simulink library "downlink_4c2t_cordic_lib"  (Simulink 8.7)
settings: Solver=ode45  StartTime=0.0  StopTime=10.0  RelTol=1e-3
undefined symbols (not defined in the file or in its folder): evalAionMaskParam, primtype, value
undefined symbols (not defined in the file): nco_angle_bits, nco_out_bits
libraries: DSPBAPrim x55, CORDIC_lib x35
settings Model: Creator=bcope  LastModifiedBy=5g

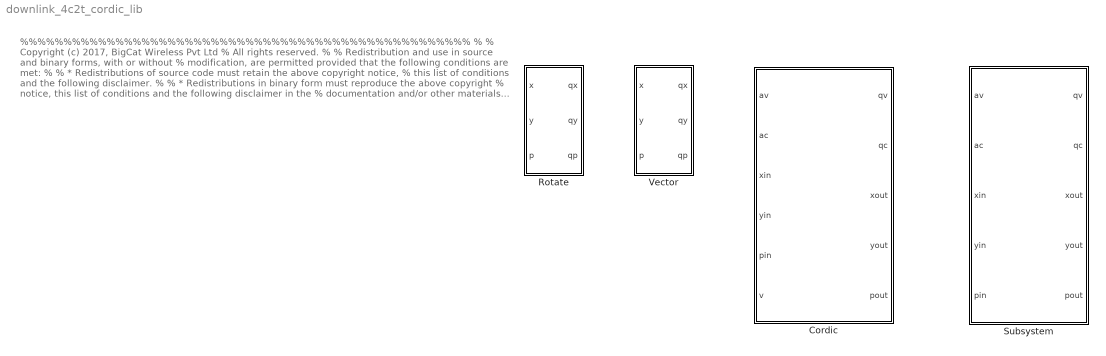
== system downlink_4c2t_cordic_lib ==
  note: %%%%%%%%%%%%%%%%%%%%%%%%%%%%%%%%%%%%%%%%%%%%%%%%%%%%
      |  %
      |  % Copyright (c) 2017, BigCat Wireless Pvt Ltd
      |  % All rights reserved.
      |  %
      |  % Redistribution and use in source and binary forms, with or without
      |  % modification, are permitted provided that the following conditions are met:
      |  %
      |  %     * Redistributions of source code must retain the above copyright notice,
      |  %       this list of conditions and the following disclaimer.
      |  %
      |  %     * Redistributions in binary form must reproduce the above copyright
      |  %       notice, this list of conditions and the following disclaimer in the
      |  %       documentation and/or other materials provided with the distribution.
      |  %
      |  %     * Neither the name of the copyright holder nor the names of its contributors
      |  %       may be used to endorse or promote products derived from this software
      |  %       without specific prior written permission.
      |  %
      |  %
      |  %
      |  % THIS SOFTWARE IS PROVIDED BY THE COPYRIGHT HOLDERS AND CONTRIBUTORS "AS IS"
      |  % AND ANY EXPRESS OR IMPLIED WARRANTIES, INCLUDING, BUT NOT LIMITED TO, THE
      |  % IMPLIED WARRANTIES OF MERCHANTABILITY AND FITNESS FOR A PARTICULAR PURPOSE ARE
      |  % DISCLAIMED. IN NO EVENT SHALL THE COPYRIGHT HOLDER OR CONTRIBUTORS BE LIABLE
      |  % FOR ANY DIRECT, INDIRECT, INCIDENTAL, SPECIAL, EXEMPLARY, OR CONSEQUENTIAL
      |  % DAMAGES (INCLUDING, BUT NOT LIMITED TO, PROCUREMENT OF SUBSTITUTE GOODS OR
      |  % SERVICES; LOSS OF USE, DATA, OR PROFITS; OR BUSINESS INTERRUPTION) HOWEVER
      |  % CAUSED AND ON ANY THEORY OF LIABILITY, WHETHER IN CONTRACT, STRICT LIABILITY,
      |  % OR TORT (INCLUDING NEGLIGENCE OR OTHERWISE) ARISING IN ANY WAY OUT OF THE USE
      |  % OF THIS SOFTWARE, EVEN IF ADVISED OF THE POSSIBILITY OF SUCH DAMAGE.
      |  %
      |   %%%%%%%%%%%%%%%%%%%%%%%%%%%%%%%%%%%%%%%%%%%%%%%%%%%%%
  Cordic : Subsystem  mask(CORDIC range -pi/2 to pi/2){stages=16, angle_bits=16, angle_frac_bits=14, xy_bits=16, xy_frac_bits=14}
      mask prompts: angle_bits "Angle bits"; angle_frac_bits "Angle fractional bits"; xy_bits "XY bits"; xy_frac_bits "XY fractional bits"
      mask help:
      | Primitive block implementation of CORDIC.
      | Range -pi/2 to pi/2
      |
      | See "Help" for information on parameter selection.
      mask init:
      | setup_cordic_block(stages, angle_bits, angle_frac_bits, xy_bits, xy_frac_bits);
      mask Help:
      | By default it is expected that stages = angle_bits = xy_bits also that
      | angle_frac_bits = angle_bits-2 (i.e. 2 integer angle bits)
      | 
      | It is assumed that stages <= angle_bits and stages <= xy_bits
      | 
      | Parameter description:
      | 
      | Stages (stages)
      | Number of CORDIC stages
      | Note counting starts at zero so "iterations = stages+1"
      | 
      | Angle bits (angle_bits)
      | Number of bits used to represent the angle, data format is "sfix"
      | 
      | Angle fractional bits (angle_frac_bits)
      | Number of angle bits which are fractional
      | Angle format will be "sfix[angle_bits]_[angle_frac_bits]"
      | 
      | XY bits (xy_bits)
      | Number of bits used to represent inputs x,y, data format is "sfix"
      | 
      | XY fractional bits (xy_frac_bits)
      | Number of x,y bits which are fractional
      | Format will be "sfix[xy_bits]_[xy_frac_bits]"
      | 
      | 
      | For more information on CORDIC see the following paper (from which this
      | implementation was created):
      | 
      | "A survey of CORDIC algorithms for FPGAs"
      | Ray Andraka, FPGA '98
      mask Display:
      | % calculate gain
      | gain = 1;
      | for i=0:stages
      |     gain = gain*(sqrt((1+2^(-2*i))));
      | end
      | color('w');image(imread('dspba_prim.jpg'));
      | fprintf('CORDIC\n(pi/2 to -pi/2)\ngain=%1.4f\niterations=%i',gain,stages+1);
      | 
      | port_label('input',1,'v_in');
      | port_label('input',2,'c_in');
      | port_label('input',3,'x_in');
      | port_label('input',4,'y_in');
      | port_label('input',5,'p_in');
      | port_label('input',6,'mode');
      | port_label('output',1,'v_out');
      | port_label('output',2,'c_out');
      | port_label('output',3,'x_out');
      | port_label('output',4,'y_out');
      | port_label('output',5,'p_out');
  Rotate : Subsystem  mask{stage=0, angle_bits=16, angle_frac_bits=14, xy_bits=16, xy_frac_bits=14}
      mask prompts: angle_bits "Angle bit width"; angle_frac_bits "Angle fractional bits"; xy_bits "XY bit width"; xy_frac_bits "XY fractional bits"
  Subsystem : Subsystem  mask{stages=nco_angle_bits, angle_bits=nco_angle_bits, angle_frac_bits=nco_angle_bits-3, xy_bits=nco_out_bits, xy_frac_bits=nco_out_bits-2}
      mask prompts: angle_bits "Angle bits"; angle_frac_bits "Angle fractional bits"; xy_bits "XY bits"; xy_frac_bits "XY fractional bits"
      mask init:
      | sys = gcb;
      | 
      | % error trapping
      | if (angle_bits-angle_frac_bits)<3
      |     fprintf(['Warning (' sys ') not sufficient angle integer bits to represent full angle swing (-pi to pi)']);
      | end
      | 
      | if angle_bits < stages 
      |     fprintf(['Warning (' sys ') #angle bits < stages behaviour may be unexpected']);
      | end
      | 
      | if xy_bits < stages 
      |     fprintf(['Warning (' sys ') #xy bits < stages behaviour may be unexpected']);
      | end
      mask Display:
      | % calculate gain
      | gain = 1;
      | for i=0:stages
      |     gain = gain*(sqrt((1+2^(-2*i))));
      | end
      | color('w');image(imread('dspba_prim.jpg'));
      | fprintf('CORDIC\nRotate\n(pi to -pi)\ngain=%1.4f\niterations=%i',gain,stages+1);
      | port_label('input',1,'v_in');
      | port_label('input',2,'c_in');
      | port_label('input',3,'x_in');
      | port_label('input',4,'y_in');
      | port_label('input',5,'p_in');
      | port_label('output',1,'v_out');
      | port_label('output',2,'c_out');
      | port_label('output',3,'x_out');
      | port_label('output',4,'y_out');
      | port_label('output',5,'p_out');
  Vector : Subsystem  mask{stage=0, angle_bits=16, angle_frac_bits=14, xy_bits=16, xy_frac_bits=14}
      mask prompts: angle_bits "Angle bits"; angle_frac_bits "Angle fractional bits"; xy_bits "XY bits"; xy_frac_bits "XY fractional bits"

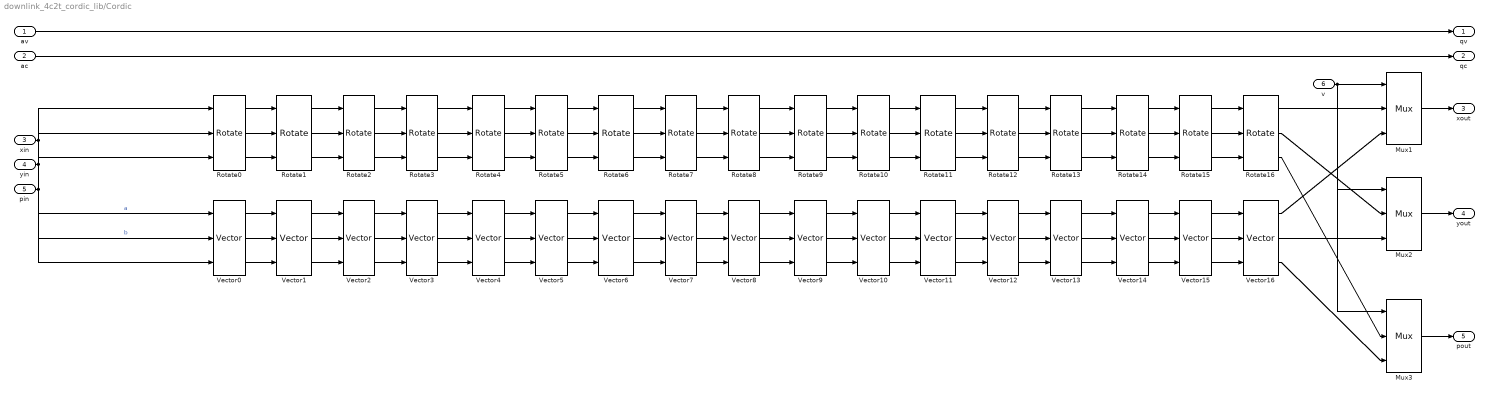
== system downlink_4c2t_cordic_lib/Cordic ==
  av : Inport
  ac : Inport  Port=2
  xin : Inport  Port=3
  yin : Inport  Port=4
  pin : Inport  Port=5
  v : Inport  Port=6
  Mux1 : DSPBAPrim/Mux  primtype=mux  nInputs=evalAionMaskParam(gcb,'value',1)+1  nOutputs=1  omode=Inherit via internal rule  otype=sfix(16)  scale=2^-15  rndmethod=Unbiased  factor=1  satmethod=Symmetric  shift_vec=[0 1 2 -1]  value=2  inPortNames=['s'; 'd0'; 'd1'; 'd2'; 'd3'; 'd4'; 'd5'; 'd6'; 'd7'; 'd8'; 'd9';]  outPortNames=[' ']  dspbaimage=dspba_prim.jpg  text=fprintf('%s', primtype);  style=Optimised  visibilities=1032  version=20131025
  Mux2 : DSPBAPrim/Mux  primtype=mux  nInputs=evalAionMaskParam(gcb,'value',1)+1  nOutputs=1  omode=Inherit via internal rule  otype=sfix(16)  scale=2^-15  rndmethod=Unbiased  factor=1  satmethod=Symmetric  shift_vec=[0 1 2 -1]  value=2  inPortNames=['s'; 'd0'; 'd1'; 'd2'; 'd3'; 'd4'; 'd5'; 'd6'; 'd7'; 'd8'; 'd9';]  outPortNames=[' ']  dspbaimage=dspba_prim.jpg  text=fprintf('%s', primtype);  style=Optimised  visibilities=1032  version=20131025
  Mux3 : DSPBAPrim/Mux  primtype=mux  nInputs=evalAionMaskParam(gcb,'value',1)+1  nOutputs=1  omode=Inherit via internal rule  otype=sfix(16)  scale=2^-15  rndmethod=Unbiased  factor=1  satmethod=Symmetric  shift_vec=[0 1 2 -1]  value=2  inPortNames=['s'; 'd0'; 'd1'; 'd2'; 'd3'; 'd4'; 'd5'; 'd6'; 'd7'; 'd8'; 'd9';]  outPortNames=[' ']  dspbaimage=dspba_prim.jpg  text=fprintf('%s', primtype);  style=Optimised  visibilities=1032  version=20131025
  Rotate0 : CORDIC_lib/Rotate  stage=0  angle_bits=16  angle_frac_bits=14  xy_bits=16  xy_frac_bits=14
  Rotate1 : CORDIC_lib/Rotate  stage=1  angle_bits=16  angle_frac_bits=14  xy_bits=16  xy_frac_bits=14
  Rotate10 : CORDIC_lib/Rotate  stage=10  angle_bits=16  angle_frac_bits=14  xy_bits=16  xy_frac_bits=14
  Rotate11 : CORDIC_lib/Rotate  stage=11  angle_bits=16  angle_frac_bits=14  xy_bits=16  xy_frac_bits=14
  Rotate12 : CORDIC_lib/Rotate  stage=12  angle_bits=16  angle_frac_bits=14  xy_bits=16  xy_frac_bits=14
  Rotate13 : CORDIC_lib/Rotate  stage=13  angle_bits=16  angle_frac_bits=14  xy_bits=16  xy_frac_bits=14
  Rotate14 : CORDIC_lib/Rotate  stage=14  angle_bits=16  angle_frac_bits=14  xy_bits=16  xy_frac_bits=14
  Rotate15 : CORDIC_lib/Rotate  stage=15  angle_bits=16  angle_frac_bits=14  xy_bits=16  xy_frac_bits=14
  Rotate16 : CORDIC_lib/Rotate  stage=16  angle_bits=16  angle_frac_bits=14  xy_bits=16  xy_frac_bits=14
  Rotate2 : CORDIC_lib/Rotate  stage=2  angle_bits=16  angle_frac_bits=14  xy_bits=16  xy_frac_bits=14
  Rotate3 : CORDIC_lib/Rotate  stage=3  angle_bits=16  angle_frac_bits=14  xy_bits=16  xy_frac_bits=14
  Rotate4 : CORDIC_lib/Rotate  stage=4  angle_bits=16  angle_frac_bits=14  xy_bits=16  xy_frac_bits=14
  Rotate5 : CORDIC_lib/Rotate  stage=5  angle_bits=16  angle_frac_bits=14  xy_bits=16  xy_frac_bits=14
  Rotate6 : CORDIC_lib/Rotate  stage=6  angle_bits=16  angle_frac_bits=14  xy_bits=16  xy_frac_bits=14
  Rotate7 : CORDIC_lib/Rotate  stage=7  angle_bits=16  angle_frac_bits=14  xy_bits=16  xy_frac_bits=14
  Rotate8 : CORDIC_lib/Rotate  stage=8  angle_bits=16  angle_frac_bits=14  xy_bits=16  xy_frac_bits=14
  Rotate9 : CORDIC_lib/Rotate  stage=9  angle_bits=16  angle_frac_bits=14  xy_bits=16  xy_frac_bits=14
  Vector0 : CORDIC_lib/Vector  stage=0  angle_bits=16  angle_frac_bits=14  xy_bits=16  xy_frac_bits=14
  Vector1 : CORDIC_lib/Vector  stage=1  angle_bits=16  angle_frac_bits=14  xy_bits=16  xy_frac_bits=14
  Vector10 : CORDIC_lib/Vector  stage=10  angle_bits=16  angle_frac_bits=14  xy_bits=16  xy_frac_bits=14
  Vector11 : CORDIC_lib/Vector  stage=11  angle_bits=16  angle_frac_bits=14  xy_bits=16  xy_frac_bits=14
  Vector12 : CORDIC_lib/Vector  stage=12  angle_bits=16  angle_frac_bits=14  xy_bits=16  xy_frac_bits=14
  Vector13 : CORDIC_lib/Vector  stage=13  angle_bits=16  angle_frac_bits=14  xy_bits=16  xy_frac_bits=14
  Vector14 : CORDIC_lib/Vector  stage=14  angle_bits=16  angle_frac_bits=14  xy_bits=16  xy_frac_bits=14
  Vector15 : CORDIC_lib/Vector  stage=15  angle_bits=16  angle_frac_bits=14  xy_bits=16  xy_frac_bits=14
  Vector16 : CORDIC_lib/Vector  stage=16  angle_bits=16  angle_frac_bits=14  xy_bits=16  xy_frac_bits=14
  Vector2 : CORDIC_lib/Vector  stage=2  angle_bits=16  angle_frac_bits=14  xy_bits=16  xy_frac_bits=14
  Vector3 : CORDIC_lib/Vector  stage=3  angle_bits=16  angle_frac_bits=14  xy_bits=16  xy_frac_bits=14
  Vector4 : CORDIC_lib/Vector  stage=4  angle_bits=16  angle_frac_bits=14  xy_bits=16  xy_frac_bits=14
  Vector5 : CORDIC_lib/Vector  stage=5  angle_bits=16  angle_frac_bits=14  xy_bits=16  xy_frac_bits=14
  Vector6 : CORDIC_lib/Vector  stage=6  angle_bits=16  angle_frac_bits=14  xy_bits=16  xy_frac_bits=14
  Vector7 : CORDIC_lib/Vector  stage=7  angle_bits=16  angle_frac_bits=14  xy_bits=16  xy_frac_bits=14
  Vector8 : CORDIC_lib/Vector  stage=8  angle_bits=16  angle_frac_bits=14  xy_bits=16  xy_frac_bits=14
  Vector9 : CORDIC_lib/Vector  stage=9  angle_bits=16  angle_frac_bits=14  xy_bits=16  xy_frac_bits=14
  qv : Outport
  qc : Outport  Port=2
  xout : Outport  Port=3
  yout : Outport  Port=4
  pout : Outport  Port=5
  wires:
  av/1 -> qv/1
  ac/1 -> qc/1
  xin/1 -> Rotate0/1, Vector0/1  "a"
  yin/1 -> Rotate0/2, Vector0/2  "b"
  pin/1 -> Rotate0/3, Vector0/3
  Rotate0/1 -> Rotate1/1
  Vector0/1 -> Vector1/1
  Rotate0/2 -> Rotate1/2
  Vector0/2 -> Vector1/2
  Rotate0/3 -> Rotate1/3
  Vector0/3 -> Vector1/3
  Rotate1/1 -> Rotate2/1
  Vector1/1 -> Vector2/1
  Rotate1/2 -> Rotate2/2
  Vector1/2 -> Vector2/2
  Rotate1/3 -> Rotate2/3
  Vector1/3 -> Vector2/3
  Rotate2/1 -> Rotate3/1
  Vector2/1 -> Vector3/1
  Rotate2/2 -> Rotate3/2
  Vector2/2 -> Vector3/2
  Rotate2/3 -> Rotate3/3
  Vector2/3 -> Vector3/3
  Rotate3/1 -> Rotate4/1
  Vector3/1 -> Vector4/1
  Rotate3/2 -> Rotate4/2
  Vector3/2 -> Vector4/2
  Rotate3/3 -> Rotate4/3
  Vector3/3 -> Vector4/3
  Rotate4/1 -> Rotate5/1
  Vector4/1 -> Vector5/1
  Rotate4/2 -> Rotate5/2
  Vector4/2 -> Vector5/2
  Rotate4/3 -> Rotate5/3
  Vector4/3 -> Vector5/3
  Rotate5/1 -> Rotate6/1
  Vector5/1 -> Vector6/1
  Rotate5/2 -> Rotate6/2
  Vector5/2 -> Vector6/2
  Rotate5/3 -> Rotate6/3
  Vector5/3 -> Vector6/3
  Rotate6/1 -> Rotate7/1
  Vector6/1 -> Vector7/1
  Rotate6/2 -> Rotate7/2
  Vector6/2 -> Vector7/2
  Rotate6/3 -> Rotate7/3
  Vector6/3 -> Vector7/3
  Rotate7/1 -> Rotate8/1
  Vector7/1 -> Vector8/1
  Rotate7/2 -> Rotate8/2
  Vector7/2 -> Vector8/2
  Rotate7/3 -> Rotate8/3
  Vector7/3 -> Vector8/3
  Rotate8/1 -> Rotate9/1
  Vector8/1 -> Vector9/1
  Rotate8/2 -> Rotate9/2
  Vector8/2 -> Vector9/2
  Rotate8/3 -> Rotate9/3
  Vector8/3 -> Vector9/3
  Rotate9/1 -> Rotate10/1
  Vector9/1 -> Vector10/1
  Rotate9/2 -> Rotate10/2
  Vector9/2 -> Vector10/2
  Rotate9/3 -> Rotate10/3
  Vector9/3 -> Vector10/3
  Rotate10/1 -> Rotate11/1
  Vector10/1 -> Vector11/1
  Rotate10/2 -> Rotate11/2
  Vector10/2 -> Vector11/2
  Rotate10/3 -> Rotate11/3
  Vector10/3 -> Vector11/3
  Rotate11/1 -> Rotate12/1
  Vector11/1 -> Vector12/1
  Rotate11/2 -> Rotate12/2
  Vector11/2 -> Vector12/2
  Rotate11/3 -> Rotate12/3
  Vector11/3 -> Vector12/3
  Rotate12/1 -> Rotate13/1
  Vector12/1 -> Vector13/1
  Rotate12/2 -> Rotate13/2
  Vector12/2 -> Vector13/2
  Rotate12/3 -> Rotate13/3
  Vector12/3 -> Vector13/3
  Rotate13/1 -> Rotate14/1
  Vector13/1 -> Vector14/1
  Rotate13/2 -> Rotate14/2
  Vector13/2 -> Vector14/2
  Rotate13/3 -> Rotate14/3
  Vector13/3 -> Vector14/3
  Rotate14/1 -> Rotate15/1
  Vector14/1 -> Vector15/1
  Rotate14/2 -> Rotate15/2
  Vector14/2 -> Vector15/2
  Rotate14/3 -> Rotate15/3
  Vector14/3 -> Vector15/3
  Rotate15/1 -> Rotate16/1
  Vector15/1 -> Vector16/1
  Rotate15/2 -> Rotate16/2
  Vector15/2 -> Vector16/2
  Rotate15/3 -> Rotate16/3
  Vector15/3 -> Vector16/3
  v/1 -> Mux1/1, Mux2/1, Mux3/1
  Rotate16/1 -> Mux1/2
  Vector16/1 -> Mux1/3
  Rotate16/2 -> Mux2/2
  Vector16/2 -> Mux2/3
  Rotate16/3 -> Mux3/2
  Vector16/3 -> Mux3/3
  Mux1/1 -> xout/1
  Mux2/1 -> yout/1
  Mux3/1 -> pout/1

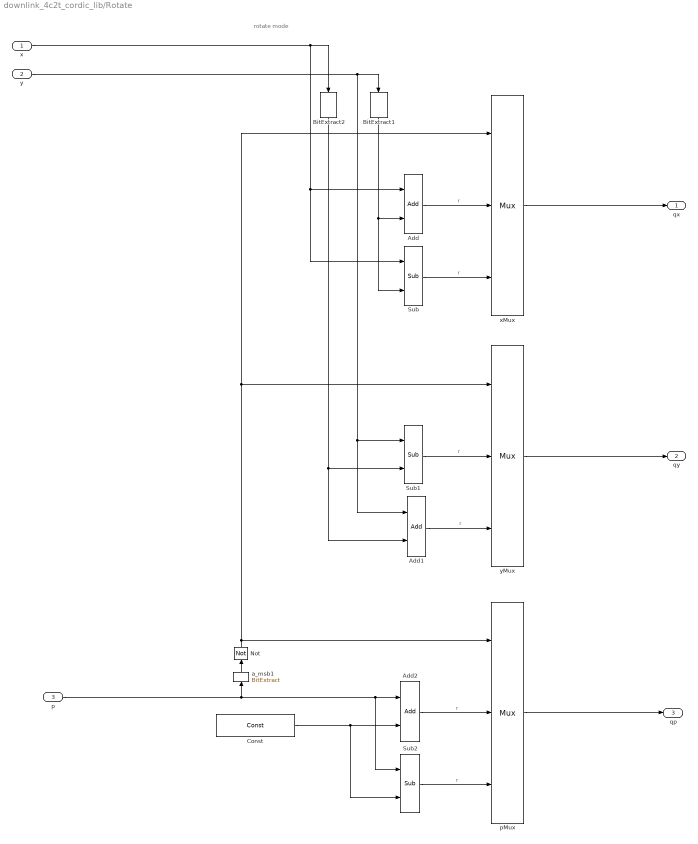
== system downlink_4c2t_cordic_lib/Rotate ==
  note: rotate mode
  x : Inport
  y : Inport  Port=2
  p : Inport  Port=3
  Add : DSPBAPrim/Add  primtype=add  nInputs=evalAionMaskParam(gcb,'value',1)  nOutputs=1  omode=Inherit via internal rule  otype=sfix(16)  scale=2^-15  rndmethod=Unbiased  factor=1  satmethod=Symmetric  shift_vec=[0 1 2 -1]  value=2  inPortNames=[' '; ' ';]  outPortNames=[' ']  dspbaimage=dspba_prim.jpg  text=fprintf('+');  style=Optimised  visibilities=1032  genFPC=off  floatRounding=correct  advOptions=[]  version=20130821
  Add1 : DSPBAPrim/Add  primtype=add  nInputs=evalAionMaskParam(gcb,'value',1)  nOutputs=1  omode=Inherit via internal rule  otype=sfix(16)  scale=2^-15  rndmethod=Unbiased  factor=1  satmethod=Symmetric  shift_vec=[0 1 2 -1]  value=2  inPortNames=[' '; ' ';]  outPortNames=[' ']  dspbaimage=dspba_prim.jpg  text=fprintf('+');  style=Optimised  visibilities=1032  genFPC=off  floatRounding=correct  advOptions=[]  version=20130821
  Add2 : DSPBAPrim/Add  primtype=add  nInputs=evalAionMaskParam(gcb,'value',1)  nOutputs=1  omode=Inherit via internal rule  otype=sfix(16)  scale=2^-15  rndmethod=Unbiased  factor=1  satmethod=Symmetric  shift_vec=[0 1 2 -1]  value=2  inPortNames=[' '; ' ';]  outPortNames=[' ']  dspbaimage=dspba_prim.jpg  text=fprintf('+');  style=Optimised  visibilities=1032  genFPC=off  floatRounding=correct  advOptions=[]  version=20130821
  BitExtract1 : DSPBAPrim/BitExtract  primtype=bitextract  nInputs=1  nOutputs=1  omode=Specify via dialog  otype=sfix(xy_bits)  scale=2^-(xy_frac_bits)  rndmethod=Unbiased  factor=1  satmethod=Symmetric  shift_vec=[0 1 2 -1]  value=stage  inPortNames=[' '; ' ';]  outPortNames=[' ']  dspbaimage=dspba_prim.jpg  text=fprintf('..%d', value);  style=Optimised  visibilities=8 + 1024  version=20090407
  BitExtract2 : DSPBAPrim/BitExtract  primtype=bitextract  nInputs=1  nOutputs=1  omode=Specify via dialog  otype=sfix(xy_bits)  scale=2^-(xy_frac_bits)  rndmethod=Unbiased  factor=1  satmethod=Symmetric  shift_vec=[0 1 2 -1]  value=stage  inPortNames=[' '; ' ';]  outPortNames=[' ']  dspbaimage=dspba_prim.jpg  text=fprintf('..%d', value);  style=Optimised  visibilities=8 + 1024  version=20090407
  Const : DSPBAPrim/Const  primtype=const  nInputs=0  nOutputs=1  omode=Specify via dialog  otype=sfix(angle_bits)  scale=2^-(angle_frac_bits)  rndmethod=Unbiased  factor=1  satmethod=Symmetric  shift_vec=[0 1 2 -1]  value=atan(2^-stage)  inPortNames=['+'; '+';]  outPortNames=[' ']  dspbaimage=dspba_prim.jpg  text=fprintf('%g', value);  style=Optimised  visibilities=8 + 1024  floatPrecision=float32_m23  version=20120820
  Not : DSPBAPrim/Not  primtype=not  nInputs=1  nOutputs=1  omode=Inherit via internal rule  otype=sfix(16)  scale=2^-15  rndmethod=Unbiased  factor=1  satmethod=Symmetric  shift_vec=[0 1 2 -1]  value=0  inPortNames=[' '; ' ';]  outPortNames=[' ']  dspbaimage=dspba_prim.jpg  text=fprintf('~');  style=Optimised  visibilities=8  version=20090407
  Sub : DSPBAPrim/Sub  primtype=sub  nInputs=2  nOutputs=1  omode=Inherit via internal rule  otype=sfix(16)  scale=2^-15  rndmethod=Unbiased  factor=1  satmethod=Symmetric  shift_vec=[0 1 2 -1]  value=0  inPortNames=['+'; '-';]  outPortNames=[' ']  dspbaimage=dspba_prim.jpg  text=fprintf('-');  style=Optimised  visibilities=8  floatRounding=correct  advOptions=[]  version=20130115
  Sub1 : DSPBAPrim/Sub  primtype=sub  nInputs=2  nOutputs=1  omode=Inherit via internal rule  otype=sfix(16)  scale=2^-15  rndmethod=Unbiased  factor=1  satmethod=Symmetric  shift_vec=[0 1 2 -1]  value=0  inPortNames=['+'; '-';]  outPortNames=[' ']  dspbaimage=dspba_prim.jpg  text=fprintf('-');  style=Optimised  visibilities=8  floatRounding=correct  advOptions=[]  version=20130115
  Sub2 : DSPBAPrim/Sub  primtype=sub  nInputs=2  nOutputs=1  omode=Inherit via internal rule  otype=sfix(16)  scale=2^-15  rndmethod=Unbiased  factor=1  satmethod=Symmetric  shift_vec=[0 1 2 -1]  value=0  inPortNames=['+'; '-';]  outPortNames=[' ']  dspbaimage=dspba_prim.jpg  text=fprintf('-');  style=Optimised  visibilities=8  floatRounding=correct  advOptions=[]  version=20130115
  a_msb1 : DSPBAPrim/BitExtract  primtype=bitextract  nInputs=1  nOutputs=1  omode=Specify via dialog  otype=ufix(1)  scale=2^-0  rndmethod=Unbiased  factor=1  satmethod=Symmetric  shift_vec=[0 1 2 -1]  value=angle_bits-1  inPortNames=[' '; ' ';]  outPortNames=[' ']  dspbaimage=dspba_prim.jpg  text=fprintf('..%d', value);  style=Optimised  visibilities=8 + 1024  version=20090407
  pMux : DSPBAPrim/Mux  primtype=mux  nInputs=evalAionMaskParam(gcb,'value',1)+1  nOutputs=1  omode=Inherit via internal rule  otype=sfix(16)  scale=2^-15  rndmethod=Unbiased  factor=1  satmethod=Symmetric  shift_vec=[0 1 2 -1]  value=2  inPortNames=['s'; '0'; '1'; '2'; '3'; '4'; '5'; '6'; '7'; '8']  outPortNames=[' ']  dspbaimage=dspba_prim.jpg  text=fprintf('%s', primtype);  style=Optimised  visibilities=1032  version=20131025
  xMux : DSPBAPrim/Mux  primtype=mux  nInputs=evalAionMaskParam(gcb,'value',1)+1  nOutputs=1  omode=Inherit via internal rule  otype=sfix(16)  scale=2^-15  rndmethod=Unbiased  factor=1  satmethod=Symmetric  shift_vec=[0 1 2 -1]  value=2  inPortNames=['s'; '0'; '1'; '2'; '3'; '4'; '5'; '6'; '7'; '8']  outPortNames=[' ']  dspbaimage=dspba_prim.jpg  text=fprintf('%s', primtype);  style=Optimised  visibilities=1032  version=20131025
  yMux : DSPBAPrim/Mux  primtype=mux  nInputs=evalAionMaskParam(gcb,'value',1)+1  nOutputs=1  omode=Inherit via internal rule  otype=sfix(16)  scale=2^-15  rndmethod=Unbiased  factor=1  satmethod=Symmetric  shift_vec=[0 1 2 -1]  value=2  inPortNames=['s'; '0'; '1'; '2'; '3'; '4'; '5'; '6'; '7'; '8']  outPortNames=[' ']  dspbaimage=dspba_prim.jpg  text=fprintf('%s', primtype);  style=Optimised  visibilities=1032  version=20131025
  qx : Outport
  qy : Outport  Port=2
  qp : Outport  Port=3
  wires:
  BitExtract2/1 -> Add1/2, Sub1/2
  BitExtract1/1 -> Sub/2, Add/2
  Const/1 -> Sub2/2, Add2/2
  p/1 -> Sub2/1, Add2/1, a_msb1/1
  pMux/1 -> qp/1
  Sub2/1 -> pMux/3  "r"
  Add2/1 -> pMux/2  "r"
  yMux/1 -> qy/1
  Add1/1 -> yMux/3  "r"
  Sub1/1 -> yMux/2  "r"
  xMux/1 -> qx/1
  Sub/1 -> xMux/3  "r"
  Add/1 -> xMux/2  "r"
  x/1 -> BitExtract2/1, Sub/1, Add/1
  y/1 -> BitExtract1/1, Add1/1, Sub1/1
  a_msb1/1 -> Not/1
  Not/1 -> xMux/1, yMux/1, pMux/1

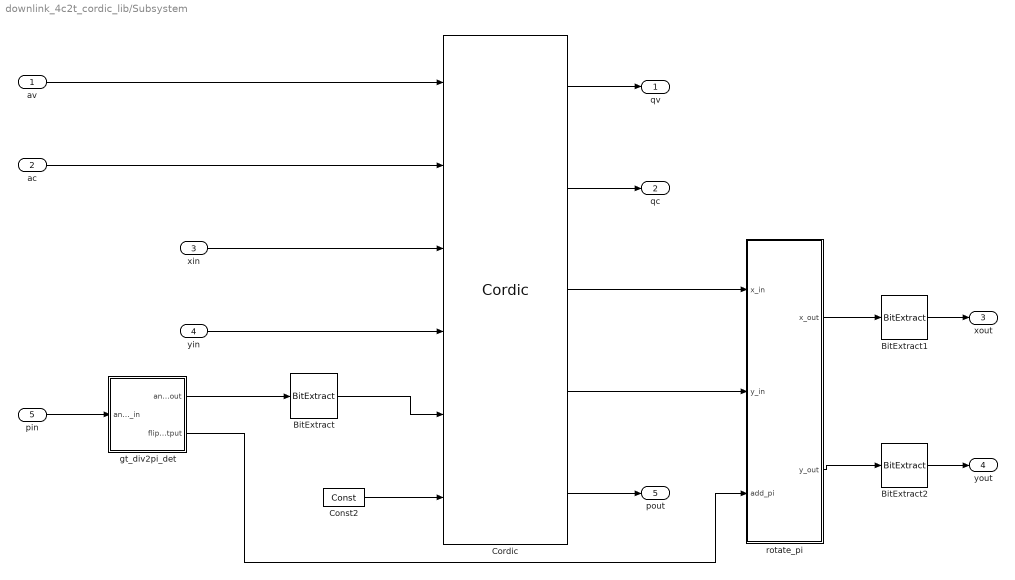
== system downlink_4c2t_cordic_lib/Subsystem ==
  av : Inport
  ac : Inport  Port=2
  xin : Inport  Port=3
  yin : Inport  Port=4
  pin : Inport  Port=5
  BitExtract : DSPBAPrim/BitExtract  primtype=bitextract  nInputs=1  nOutputs=1  omode=Specify via dialog  otype=sfix(angle_bits-1)  scale=2^-angle_frac_bits  rndmethod=Unbiased  factor=1  satmethod=Symmetric  shift_vec=[0 1 2 -1]  value=0  inPortNames=[' '; ' ';]  outPortNames=[' ']  dspbaimage=dspba_prim.jpg  text=fprintf('..%d', value);  style=Optimised  visibilities=8 + 1024  version=20090407
  BitExtract1 : DSPBAPrim/BitExtract  primtype=bitextract  nInputs=1  nOutputs=1  omode=Specify via dialog  otype=sfix(xy_bits)  scale=2^-xy_frac_bits  rndmethod=Unbiased  factor=1  satmethod=Symmetric  shift_vec=[0 1 2 -1]  value=0  inPortNames=[' '; ' ';]  outPortNames=[' ']  dspbaimage=dspba_prim.jpg  text=fprintf('..%d', value);  style=Optimised  visibilities=8 + 1024  version=20090407
  BitExtract2 : DSPBAPrim/BitExtract  primtype=bitextract  nInputs=1  nOutputs=1  omode=Specify via dialog  otype=sfix(xy_bits)  scale=2^-xy_frac_bits  rndmethod=Unbiased  factor=1  satmethod=Symmetric  shift_vec=[0 1 2 -1]  value=0  inPortNames=[' '; ' ';]  outPortNames=[' ']  dspbaimage=dspba_prim.jpg  text=fprintf('..%d', value);  style=Optimised  visibilities=8 + 1024  version=20090407
  Const2 : DSPBAPrim/Const  primtype=const  nInputs=0  nOutputs=1  omode=Specify via dialog  otype=uint(1)  scale=2^0  rndmethod=Unbiased  factor=1  satmethod=Symmetric  shift_vec=[0 1 2 -1]  value=1  inPortNames=['+'; '+';]  outPortNames=[' ']  dspbaimage=dspba_prim.jpg  text=fprintf('%s', num2str(value));  style=Optimised  visibilities=8 + 1024  floatPrecision=float32_m23  version=20120820
  Cordic : CORDIC_lib/Cordic  stages=stages  angle_bits=angle_bits-1  angle_frac_bits=angle_frac_bits  xy_bits=xy_bits  xy_frac_bits=xy_frac_bits
  gt_div2pi_det : Subsystem  mask{angle_bits=angle_bits}
      mask prompts: angle_bits "Angle bits"
  rotate_pi : Subsystem
  qv : Outport
  qc : Outport  Port=2
  xout : Outport  Port=3
  yout : Outport  Port=4
  pout : Outport  Port=5
  wires:
  BitExtract2/1 -> yout/1
  BitExtract1/1 -> xout/1
  BitExtract/1 -> Cordic/5
  Const2/1 -> Cordic/6
  gt_div2pi_det/2(flip_output) -> rotate_pi/3(add_pi)
  rotate_pi/2(y_out) -> BitExtract2/1
  rotate_pi/1(x_out) -> BitExtract1/1
  gt_div2pi_det/1(angle_out) -> BitExtract/1
  pin/1 -> gt_div2pi_det/1(angle_in)
  yin/1 -> Cordic/4
  xin/1 -> Cordic/3
  Cordic/5 -> pout/1
  Cordic/4 -> rotate_pi/2(y_in)
  Cordic/3 -> rotate_pi/1(x_in)
  Cordic/2 -> qc/1
  Cordic/1 -> qv/1
  ac/1 -> Cordic/2
  av/1 -> Cordic/1

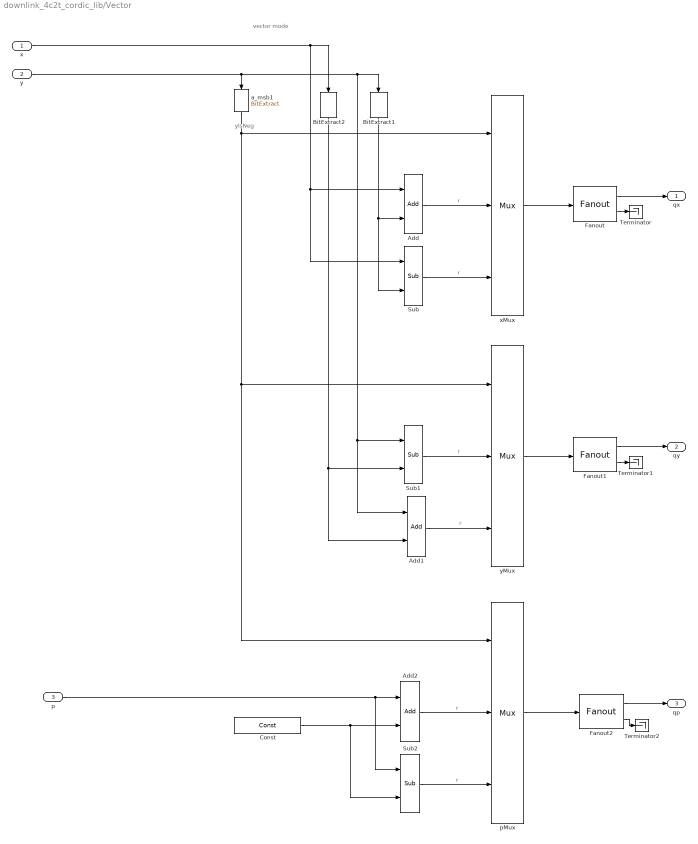
== system downlink_4c2t_cordic_lib/Vector ==
  note: vector mode
  note: yIsNeg
  x : Inport
  y : Inport  Port=2
  p : Inport  Port=3
  Add : DSPBAPrim/Add  primtype=add  nInputs=evalAionMaskParam(gcb,'value',1)  nOutputs=1  omode=Inherit via internal rule  otype=sfix(16)  scale=2^-15  rndmethod=Unbiased  factor=1  satmethod=Symmetric  shift_vec=[0 1 2 -1]  value=2  inPortNames=[' '; ' ';]  outPortNames=[' ']  dspbaimage=dspba_prim.jpg  text=fprintf('+');  style=Optimised  visibilities=1032  genFPC=off  floatRounding=correct  advOptions=[]  version=20130821
  Add1 : DSPBAPrim/Add  primtype=add  nInputs=evalAionMaskParam(gcb,'value',1)  nOutputs=1  omode=Inherit via internal rule  otype=sfix(16)  scale=2^-15  rndmethod=Unbiased  factor=1  satmethod=Symmetric  shift_vec=[0 1 2 -1]  value=2  inPortNames=[' '; ' ';]  outPortNames=[' ']  dspbaimage=dspba_prim.jpg  text=fprintf('+');  style=Optimised  visibilities=1032  genFPC=off  floatRounding=correct  advOptions=[]  version=20130821
  Add2 : DSPBAPrim/Add  primtype=add  nInputs=evalAionMaskParam(gcb,'value',1)  nOutputs=1  omode=Inherit via internal rule  otype=sfix(16)  scale=2^-15  rndmethod=Unbiased  factor=1  satmethod=Symmetric  shift_vec=[0 1 2 -1]  value=2  inPortNames=[' '; ' ';]  outPortNames=[' ']  dspbaimage=dspba_prim.jpg  text=fprintf('+');  style=Optimised  visibilities=1032  genFPC=off  floatRounding=correct  advOptions=[]  version=20130821
  BitExtract1 : DSPBAPrim/BitExtract  primtype=bitextract  nInputs=1  nOutputs=1  omode=Specify via dialog  otype=sfix(16)  scale=2^-14  rndmethod=Unbiased  factor=1  satmethod=Symmetric  shift_vec=[0 1 2 -1]  value=stage  inPortNames=[' '; ' ';]  outPortNames=[' ']  dspbaimage=dspba_prim.jpg  text=fprintf('..%d', value);  style=Optimised  visibilities=8 + 1024  version=20090407
  BitExtract2 : DSPBAPrim/BitExtract  primtype=bitextract  nInputs=1  nOutputs=1  omode=Specify via dialog  otype=sfix(16)  scale=2^-14  rndmethod=Unbiased  factor=1  satmethod=Symmetric  shift_vec=[0 1 2 -1]  value=stage  inPortNames=[' '; ' ';]  outPortNames=[' ']  dspbaimage=dspba_prim.jpg  text=fprintf('..%d', value);  style=Optimised  visibilities=8 + 1024  version=20090407
  Const : DSPBAPrim/Const  primtype=const  nInputs=0  nOutputs=1  omode=Specify via dialog  otype=sfix(16)  scale=2^-14  rndmethod=Unbiased  factor=1  satmethod=Symmetric  shift_vec=[0 1 2 -1]  value=atan(2^-stage)  inPortNames=['+'; '+';]  outPortNames=[' ']  dspbaimage=dspba_prim.jpg  text=fprintf('%g', value);  style=Optimised  visibilities=8 + 1024  floatPrecision=float32_m23  version=20120820
  Fanout : DSPBAPrim/Fanout  primtype=fanout  nInputs=1  nOutputs=evalAionMaskParam(gcb,'value',1)  omode=Inherit via internal rule  otype=sfix(16)  scale=2^-15  rndmethod=Unbiased  factor=1  satmethod=Symmetric  shift_vec=[0 1 2 -1]  value=2  inPortNames=[' '; ' ';]  outPortNames=[' ']  dspbaimage=dspba_prim.jpg  text=fprintf('fanout')  style=Optimised  visibilities=2^10+2^18  version=20150501  uninit=off
  Fanout1 : DSPBAPrim/Fanout  primtype=fanout  nInputs=1  nOutputs=evalAionMaskParam(gcb,'value',1)  omode=Inherit via internal rule  otype=sfix(16)  scale=2^-15  rndmethod=Unbiased  factor=1  satmethod=Symmetric  shift_vec=[0 1 2 -1]  value=2  inPortNames=[' '; ' ';]  outPortNames=[' ']  dspbaimage=dspba_prim.jpg  text=fprintf('fanout')  style=Optimised  visibilities=2^10+2^18  version=20150501  uninit=off
  Fanout2 : DSPBAPrim/Fanout  primtype=fanout  nInputs=1  nOutputs=evalAionMaskParam(gcb,'value',1)  omode=Inherit via internal rule  otype=sfix(16)  scale=2^-15  rndmethod=Unbiased  factor=1  satmethod=Symmetric  shift_vec=[0 1 2 -1]  value=2  inPortNames=[' '; ' ';]  outPortNames=[' ']  dspbaimage=dspba_prim.jpg  text=fprintf('fanout')  style=Optimised  visibilities=2^10+2^18  version=20150501  uninit=off
  Sub : DSPBAPrim/Sub  primtype=sub  nInputs=2  nOutputs=1  omode=Inherit via internal rule  otype=sfix(16)  scale=2^-15  rndmethod=Unbiased  factor=1  satmethod=Symmetric  shift_vec=[0 1 2 -1]  value=0  inPortNames=['+'; '-';]  outPortNames=[' ']  dspbaimage=dspba_prim.jpg  text=fprintf('-');  style=Optimised  visibilities=8  floatRounding=correct  advOptions=[]  version=20130115
  Sub1 : DSPBAPrim/Sub  primtype=sub  nInputs=2  nOutputs=1  omode=Inherit via internal rule  otype=sfix(16)  scale=2^-15  rndmethod=Unbiased  factor=1  satmethod=Symmetric  shift_vec=[0 1 2 -1]  value=0  inPortNames=['+'; '-';]  outPortNames=[' ']  dspbaimage=dspba_prim.jpg  text=fprintf('-');  style=Optimised  visibilities=8  floatRounding=correct  advOptions=[]  version=20130115
  Sub2 : DSPBAPrim/Sub  primtype=sub  nInputs=2  nOutputs=1  omode=Inherit via internal rule  otype=sfix(16)  scale=2^-15  rndmethod=Unbiased  factor=1  satmethod=Symmetric  shift_vec=[0 1 2 -1]  value=0  inPortNames=['+'; '-';]  outPortNames=[' ']  dspbaimage=dspba_prim.jpg  text=fprintf('-');  style=Optimised  visibilities=8  floatRounding=correct  advOptions=[]  version=20130115
  Terminator : Terminator
  Terminator1 : Terminator
  Terminator2 : Terminator
  a_msb1 : DSPBAPrim/BitExtract  primtype=bitextract  nInputs=1  nOutputs=1  omode=Specify via dialog  otype=ufix(1)  scale=2^-0  rndmethod=Unbiased  factor=1  satmethod=Symmetric  shift_vec=[0 1 2 -1]  value=15  inPortNames=[' '; ' ';]  outPortNames=[' ']  dspbaimage=dspba_prim.jpg  text=fprintf('..%d', value);  style=Optimised  visibilities=8 + 1024  version=20090407
  pMux : DSPBAPrim/Mux  primtype=mux  nInputs=evalAionMaskParam(gcb,'value',1)+1  nOutputs=1  omode=Inherit via internal rule  otype=sfix(16)  scale=2^-15  rndmethod=Unbiased  factor=1  satmethod=Symmetric  shift_vec=[0 1 2 -1]  value=2  inPortNames=['s'; '0'; '1'; '2'; '3'; '4'; '5'; '6'; '7'; '8']  outPortNames=[' ']  dspbaimage=dspba_prim.jpg  text=fprintf('%s', primtype);  style=Optimised  visibilities=1032  version=20131025
  xMux : DSPBAPrim/Mux  primtype=mux  nInputs=evalAionMaskParam(gcb,'value',1)+1  nOutputs=1  omode=Inherit via internal rule  otype=sfix(16)  scale=2^-15  rndmethod=Unbiased  factor=1  satmethod=Symmetric  shift_vec=[0 1 2 -1]  value=2  inPortNames=['s'; '0'; '1'; '2'; '3'; '4'; '5'; '6'; '7'; '8']  outPortNames=[' ']  dspbaimage=dspba_prim.jpg  text=fprintf('%s', primtype);  style=Optimised  visibilities=1032  version=20131025
  yMux : DSPBAPrim/Mux  primtype=mux  nInputs=evalAionMaskParam(gcb,'value',1)+1  nOutputs=1  omode=Inherit via internal rule  otype=sfix(16)  scale=2^-15  rndmethod=Unbiased  factor=1  satmethod=Symmetric  shift_vec=[0 1 2 -1]  value=2  inPortNames=['s'; '0'; '1'; '2'; '3'; '4'; '5'; '6'; '7'; '8']  outPortNames=[' ']  dspbaimage=dspba_prim.jpg  text=fprintf('%s', primtype);  style=Optimised  visibilities=1032  version=20131025
  qx : Outport
  qy : Outport  Port=2
  qp : Outport  Port=3
  wires:
  y/1 -> a_msb1/1, BitExtract1/1, Sub1/1, Add1/1
  x/1 -> Add/1, Sub/1, BitExtract2/1
  Add/1 -> xMux/2  "r"
  Sub/1 -> xMux/3  "r"
  Sub1/1 -> yMux/2  "r"
  Add1/1 -> yMux/3  "r"
  Add2/1 -> pMux/2  "r"
  Sub2/1 -> pMux/3  "r"
  p/1 -> Add2/1, Sub2/1
  Const/1 -> Add2/2, Sub2/2
  a_msb1/1 -> pMux/1, yMux/1, xMux/1
  BitExtract1/1 -> Add/2, Sub/2
  BitExtract2/1 -> Sub1/2, Add1/2
  xMux/1 -> Fanout/1
  Fanout/1 -> qx/1
  Fanout/2 -> Terminator/1
  yMux/1 -> Fanout1/1
  Fanout1/1 -> qy/1
  Fanout1/2 -> Terminator1/1
  pMux/1 -> Fanout2/1
  Fanout2/1 -> qp/1
  Fanout2/2 -> Terminator2/1

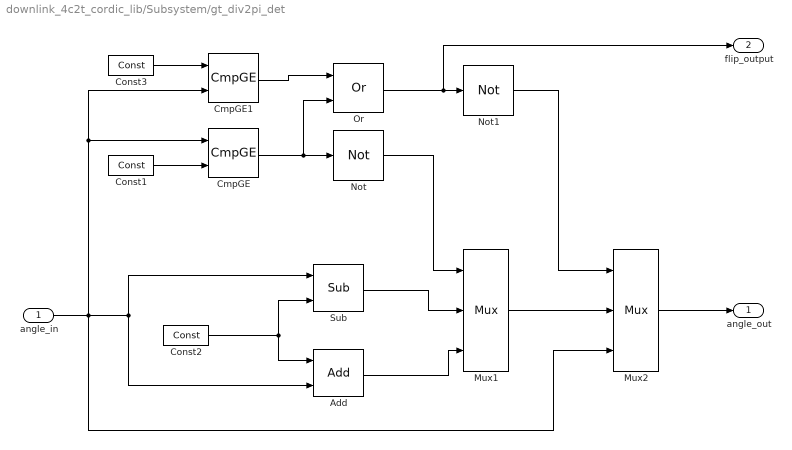
== system downlink_4c2t_cordic_lib/Subsystem/gt_div2pi_det ==
  angle_in : Inport
  Add : DSPBAPrim/Add  primtype=add  nInputs=evalAionMaskParam(gcb,'value',1)  nOutputs=1  omode=Inherit via internal rule with word growth  otype=sfix(16)  scale=2^-15  rndmethod=Unbiased  factor=1  satmethod=Symmetric  shift_vec=[0 1 2 -1]  value=2  inPortNames=[' '; ' ';]  outPortNames=[' ']  dspbaimage=dspba_prim.jpg  text=fprintf('+');  style=Optimised  visibilities=1032  version=20090731
  CmpGE : DSPBAPrim/CmpGE  primtype=cmpgte  nInputs=2  nOutputs=1  omode=boolean  otype=sfix(16)  scale=2^-15  rndmethod=Unbiased  factor=1  satmethod=Symmetric  shift_vec=[0 1 2 -1]  value=0  inPortNames=['a'; 'b';]  outPortNames=[' ']  dspbaimage=dspba_prim.jpg  text=fprintf('a>=b');  style=Optimised  visibilities=0  version=20090407
  CmpGE1 : DSPBAPrim/CmpGE  primtype=cmpgte  nInputs=2  nOutputs=1  omode=boolean  otype=sfix(16)  scale=2^-15  rndmethod=Unbiased  factor=1  satmethod=Symmetric  shift_vec=[0 1 2 -1]  value=0  inPortNames=['a'; 'b';]  outPortNames=[' ']  dspbaimage=dspba_prim.jpg  text=fprintf('a>=b');  style=Optimised  visibilities=0  version=20090407
  Const1 : DSPBAPrim/Const  primtype=const  nInputs=0  nOutputs=1  omode=Specify via dialog  otype=sfix(angle_bits)  scale=2^-(angle_bits-3)  rndmethod=Unbiased  factor=1  satmethod=Symmetric  shift_vec=[0 1 2 -1]  value=pi/2  inPortNames=['+'; '+';]  outPortNames=[' ']  dspbaimage=dspba_prim.jpg  text=fprintf('%s', num2str(value));  style=Optimised  visibilities=8 + 1024  version=20090407
  Const2 : DSPBAPrim/Const  primtype=const  nInputs=0  nOutputs=1  omode=Specify via dialog  otype=sfix(angle_bits)  scale=2^-(angle_bits-3)  rndmethod=Unbiased  factor=1  satmethod=Symmetric  shift_vec=[0 1 2 -1]  value=pi/2  inPortNames=['+'; '+';]  outPortNames=[' ']  dspbaimage=dspba_prim.jpg  text=fprintf('%s', num2str(value));  style=Optimised  visibilities=8 + 1024  version=20090407
  Const3 : DSPBAPrim/Const  primtype=const  nInputs=0  nOutputs=1  omode=Specify via dialog  otype=sfix(angle_bits)  scale=2^-(angle_bits-3)  rndmethod=Unbiased  factor=1  satmethod=Symmetric  shift_vec=[0 1 2 -1]  value=-pi/2  inPortNames=['+'; '+';]  outPortNames=[' ']  dspbaimage=dspba_prim.jpg  text=fprintf('%s', num2str(value));  style=Optimised  visibilities=8 + 1024  version=20090407
  Mux1 : DSPBAPrim/Mux  primtype=mux  nInputs=evalAionMaskParam(gcb,'value',1)+1  nOutputs=1  omode=Inherit via internal rule  otype=sfix(16)  scale=2^-15  rndmethod=Unbiased  factor=1  satmethod=Symmetric  shift_vec=[0 1 2 -1]  value=2  inPortNames=['s'; 'd0'; 'd1'; 'd2'; 'd3'; 'd4'; 'd5'; 'd6'; 'd7'; 'd8'; 'd9';]  outPortNames=[' ']  dspbaimage=dspba_prim.jpg  text=fprintf('%s', primtype);  style=Optimised  visibilities=1032  version=20090623
  Mux2 : DSPBAPrim/Mux  primtype=mux  nInputs=evalAionMaskParam(gcb,'value',1)+1  nOutputs=1  omode=Inherit via internal rule  otype=sfix(16)  scale=2^-15  rndmethod=Unbiased  factor=1  satmethod=Symmetric  shift_vec=[0 1 2 -1]  value=2  inPortNames=['s'; 'd0'; 'd1'; 'd2'; 'd3'; 'd4'; 'd5'; 'd6'; 'd7'; 'd8'; 'd9';]  outPortNames=[' ']  dspbaimage=dspba_prim.jpg  text=fprintf('%s', primtype);  style=Optimised  visibilities=1032  version=20090623
  Not : DSPBAPrim/Not  primtype=not  nInputs=1  nOutputs=1  omode=Inherit via internal rule  otype=sfix(16)  scale=2^-15  rndmethod=Unbiased  factor=1  satmethod=Symmetric  shift_vec=[0 1 2 -1]  value=0  inPortNames=[' '; ' ';]  outPortNames=[' ']  dspbaimage=dspba_prim.jpg  text=fprintf('~');  style=Optimised  visibilities=8  version=20090407
  Not1 : DSPBAPrim/Not  primtype=not  nInputs=1  nOutputs=1  omode=Inherit via internal rule  otype=sfix(16)  scale=2^-15  rndmethod=Unbiased  factor=1  satmethod=Symmetric  shift_vec=[0 1 2 -1]  value=0  inPortNames=[' '; ' ';]  outPortNames=[' ']  dspbaimage=dspba_prim.jpg  text=fprintf('~');  style=Optimised  visibilities=8  version=20090407
  Or : DSPBAPrim/Or  primtype=or  nInputs=2  nOutputs=1  omode=Inherit via internal rule  otype=sfix(16)  scale=2^-15  rndmethod=Unbiased  factor=1  satmethod=Symmetric  shift_vec=[0 1 2 -1]  value=0  inPortNames=[' '; ' '; ' '; ' '; ' '; ' '; ' '; ' '; ' '; ' '; ' '; ' '; ' '; ' '; ' '; ' '; ]  outPortNames=[' ']  dspbaimage=dspba_prim.jpg  text=fprintf('|');  style=Optimised  visibilities=8+2  version=20090407
  Sub : DSPBAPrim/Sub  primtype=sub  nInputs=2  nOutputs=1  omode=Inherit via internal rule with word growth  otype=sfix(16)  scale=2^-15  rndmethod=Unbiased  factor=1  satmethod=Symmetric  shift_vec=[0 1 2 -1]  value=0  inPortNames=['+'; '-';]  outPortNames=[' ']  dspbaimage=dspba_prim.jpg  text=fprintf('-');  style=Optimised  visibilities=8  version=20090407
  angle_out : Outport
  flip_output : Outport  Port=2
  wires:
  CmpGE1/1 -> Or/1
  Or/1 -> flip_output/1, Not1/1
  Not1/1 -> Mux2/1
  Mux1/1 -> Mux2/2
  Const3/1 -> CmpGE1/1
  Not/1 -> Mux1/1
  CmpGE/1 -> Or/2, Not/1
  Const1/1 -> CmpGE/2
  Mux2/1 -> angle_out/1
  angle_in/1 -> Mux2/3, CmpGE1/2, CmpGE/1, Add/2, Sub/1
  Add/1 -> Mux1/3
  Const2/1 -> Add/1, Sub/2
  Sub/1 -> Mux1/2

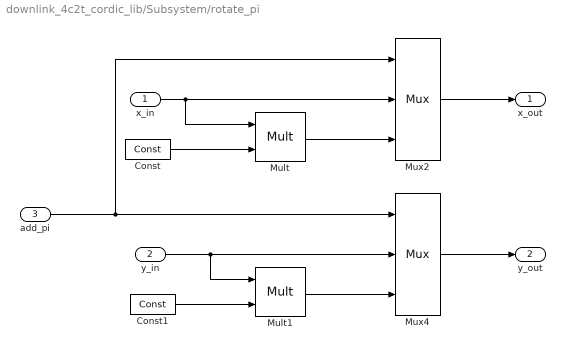
== system downlink_4c2t_cordic_lib/Subsystem/rotate_pi ==
  x_in : Inport
  y_in : Inport  Port=2
  add_pi : Inport  Port=3
  Const : DSPBAPrim/Const  primtype=const  nInputs=0  nOutputs=1  omode=Specify via dialog  otype=sfix(2)  scale=2^-0  rndmethod=Unbiased  factor=1  satmethod=Symmetric  shift_vec=[0 1 2 -1]  value=-1  inPortNames=['+'; '+';]  outPortNames=[' ']  dspbaimage=dspba_prim.jpg  text=fprintf('%s', num2str(value));  style=Optimised  visibilities=8 + 1024  version=20090407
  Const1 : DSPBAPrim/Const  primtype=const  nInputs=0  nOutputs=1  omode=Specify via dialog  otype=sfix(2)  scale=2^-0  rndmethod=Unbiased  factor=1  satmethod=Symmetric  shift_vec=[0 1 2 -1]  value=-1  inPortNames=['+'; '+';]  outPortNames=[' ']  dspbaimage=dspba_prim.jpg  text=fprintf('%s', num2str(value));  style=Optimised  visibilities=8 + 1024  version=20090407
  Mult : DSPBAPrim/Mult  primtype=mult  nInputs=2  nOutputs=1  omode=Inherit via internal rule  otype=sfix(16)  scale=2^-15  rndmethod=Unbiased  factor=1  satmethod=Symmetric  shift_vec=[0 1 2 -1]  value=0  inPortNames=[' '; ' ';]  outPortNames=[' ']  dspbaimage=dspba_prim.jpg  text=fprintf('X');  style=Optimised  visibilities=8  version=20090407
  Mult1 : DSPBAPrim/Mult  primtype=mult  nInputs=2  nOutputs=1  omode=Inherit via internal rule  otype=sfix(16)  scale=2^-15  rndmethod=Unbiased  factor=1  satmethod=Symmetric  shift_vec=[0 1 2 -1]  value=0  inPortNames=[' '; ' ';]  outPortNames=[' ']  dspbaimage=dspba_prim.jpg  text=fprintf('X');  style=Optimised  visibilities=8  version=20090407
  Mux2 : DSPBAPrim/Mux  primtype=mux  nInputs=evalAionMaskParam(gcb,'value',1)+1  nOutputs=1  omode=Inherit via internal rule  otype=sfix(16)  scale=2^-15  rndmethod=Unbiased  factor=1  satmethod=Symmetric  shift_vec=[0 1 2 -1]  value=2  inPortNames=['s'; 'd0'; 'd1'; 'd2'; 'd3'; 'd4'; 'd5'; 'd6'; 'd7'; 'd8'; 'd9';]  outPortNames=[' ']  dspbaimage=dspba_prim.jpg  text=fprintf('%s', primtype);  style=Optimised  visibilities=1032  version=20090623
  Mux4 : DSPBAPrim/Mux  primtype=mux  nInputs=evalAionMaskParam(gcb,'value',1)+1  nOutputs=1  omode=Inherit via internal rule  otype=sfix(16)  scale=2^-15  rndmethod=Unbiased  factor=1  satmethod=Symmetric  shift_vec=[0 1 2 -1]  value=2  inPortNames=['s'; 'd0'; 'd1'; 'd2'; 'd3'; 'd4'; 'd5'; 'd6'; 'd7'; 'd8'; 'd9';]  outPortNames=[' ']  dspbaimage=dspba_prim.jpg  text=fprintf('%s', primtype);  style=Optimised  visibilities=1032  version=20090623
  x_out : Outport
  y_out : Outport  Port=2
  wires:
  Const/1 -> Mult/2
  add_pi/1 -> Mux2/1, Mux4/1
  Mult1/1 -> Mux4/3
  x_in/1 -> Mult/1, Mux2/2
  Const1/1 -> Mult1/2
  y_in/1 -> Mult1/1, Mux4/2
  Mux2/1 -> x_out/1
  Mux4/1 -> y_out/1
  Mult/1 -> Mux2/3
